simulink model "systemIdentification"  (R2018a)
settings: Solver=FixedStepDiscrete  StartTime=0.0  StopTime=finalTime  FixedStep=sampleTime  RelTol=1e-3
values from neighbouring files (symbols this model uses):
  C1A = 5e-6    (= 5e-06)    [impedance_inductanceAll.m]    (also in impedance_inductancemodel.m)
  C1B = 5e-6    (= 5e-06)    [impedance_inductanceAll.m]    (also in impedance_inductancemodel.m)
  C1C = 5e-6    (= 5e-06)    [impedance_inductanceAll.m]    (also in impedance_inductancemodel.m)
  ESLA = 3e-15    [analytical.m]    (also in impedance_inductanceAll.m = 1.9e-14; impedance_inductancemodel.m = 1.9e-14)
  ESLB = 3e-15    [analytical.m]    (also in impedance_inductanceAll.m = 1.9e-14; impedance_inductancemodel.m = 1.9e-14)
  ESLC = 3e-15    [analytical.m]    (also in impedance_inductanceAll.m = 1.9e-14; impedance_inductancemodel.m = 1.9e-14)
  LA = 0.0150    (= 0.015)    [impedance_inductanceAll.m]
  LABBot = 3e-9    (= 3e-09)    [analytical.m]    (also in impedance_inductanceAll.m = 1.02e-08; impedance_inductancemodel.m = 1.02e-08)
  LABot = 3e-9    (= 3e-09)    [analytical.m]    (also in impedance_inductanceAll.m = 2.025e-08; impedance_inductancemodel.m = 2.025e-08)
  LABTop = 3e-9    (= 3e-09)    [analytical.m]    (also in impedance_inductanceAll.m = 1.83e-08; impedance_inductancemodel.m = 1.83e-08)
  LAMid = 01.30e-9    (= 1.3e-09)    [impedance_inductanceAll.m]    (also in impedance_inductancemodel.m)
  LATop = 3e-9    (= 3e-09)    [analytical.m]    (also in impedance_inductanceAll.m = 3.4e-09; impedance_inductancemodel.m = 3.4e-09)
  LB = 0.0150    (= 0.015)    [impedance_inductanceAll.m]
  LBBot = 3e-9    (= 3e-09)    [analytical.m]    (also in impedance_inductanceAll.m = 2.038e-08; impedance_inductancemodel.m = 2.038e-08)
  LBCBot = 3e-9    (= 3e-09)    [analytical.m]    (also in impedance_inductanceAll.m = 1.114e-08; impedance_inductancemodel.m = 1.114e-08)
  LBCTop = 3e-9    (= 3e-09)    [analytical.m]    (also in impedance_inductanceAll.m = 2.184e-08; impedance_inductancemodel.m = 2.184e-08)
  LBMid = 01.30e-9    (= 1.3e-09)    [impedance_inductanceAll.m]    (also in impedance_inductancemodel.m)
  LBTop = 3e-9    (= 3e-09)    [analytical.m]    (also in impedance_inductanceAll.m = 3.38e-09; impedance_inductancemodel.m = 3.38e-09)
  LC = 0.0150    (= 0.015)    [impedance_inductanceAll.m]
  LCBot = 3e-9    (= 3e-09)    [analytical.m]    (also in impedance_inductanceAll.m = 2.094e-08; impedance_inductancemodel.m = 2.094e-08)
  LCMid = 01.30e-9    (= 1.3e-09)    [impedance_inductanceAll.m]    (also in impedance_inductancemodel.m)
  LCTop = 3e-9    (= 3e-09)    [analytical.m]    (also in impedance_inductanceAll.m = 3.41e-09; impedance_inductancemodel.m = 3.41e-09)
  RA = 10    [impedance_inductanceAll.m]
  RB = 10    [impedance_inductanceAll.m]
  RC = 10    [impedance_inductanceAll.m]
  sampleTime = 1e-7    (= 1e-07)    [impedance_inductanceAll.m]
libraries: powerlib x30, dspsrcs4 x1
settings Model: Creator=enes_  LastModifiedBy=enes_

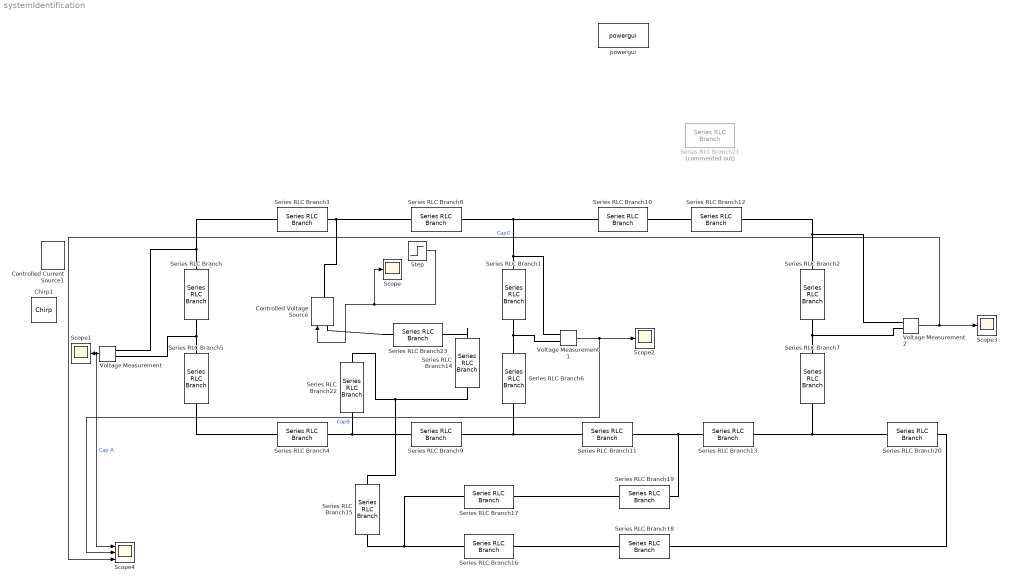
== system systemIdentification ==
  Chirp1 : dspsrcs4/Chirp  sweep=Linear  mode=Unidirectional  f0=0  f1=400000  t1=1  Tsweep=1  phase=0  Ts=sampleTime  spf=1  datatype=Double  OutputFrames=off
      settings: SourceProductName=DSP System Toolbox
  Controlled Current Source1 : powerlib/Electrical Sources/Controlled Current Source  Initialize=on  Source_Type=AC  Amplitude=0  Phase=0  Frequency=0  Measurements=None
  Controlled Voltage Source : powerlib/Electrical Sources/Controlled Voltage Source  Initialize=on  Source_Type=AC  Amplitude=0  Phase=0  Frequency=0  Measurements=None
  Scope{,1..3} (4 alike) : Scope
  Scope4 : Scope  NumInputPorts=3
  Series RLC Branch : powerlib/Elements/Series RLC Branch  LConnTagsString=__new0  RConnTagsString=__new0  BranchType=C  Resistance=1  Inductance=1e-3  SetiL0=off  InitialCurrent=0  Capacitance=C1A  Setx0=off  InitialVoltage=0  Measurements=None
  Series RLC Branch1 : powerlib/Elements/Series RLC Branch  LConnTagsString=__new0  RConnTagsString=__new0  BranchType=C  Resistance=1  Inductance=1e-3  SetiL0=off  InitialCurrent=0  Capacitance=C1B  Setx0=off  InitialVoltage=0  Measurements=None
  Series RLC Branch10 : powerlib/Elements/Series RLC Branch  LConnTagsString=__new0  RConnTagsString=__new0  BranchType=L  Resistance=1  Inductance=LBTop  SetiL0=off  InitialCurrent=0  Capacitance=1e-6  Setx0=off  InitialVoltage=0  Measurements=None
  Series RLC Branch11 : powerlib/Elements/Series RLC Branch  LConnTagsString=__new0  RConnTagsString=__new0  BranchType=L  Resistance=1  Inductance=LBBot  SetiL0=off  InitialCurrent=0  Capacitance=1e-6  Setx0=off  InitialVoltage=0  Measurements=None
  Series RLC Branch12 : powerlib/Elements/Series RLC Branch  LConnTagsString=__new0  RConnTagsString=__new0  BranchType=L  Resistance=1  Inductance=LBCTop  SetiL0=off  InitialCurrent=0  Capacitance=1e-6  Setx0=off  InitialVoltage=0  Measurements=None
  Series RLC Branch13 : powerlib/Elements/Series RLC Branch  LConnTagsString=__new0  RConnTagsString=__new0  BranchType=L  Resistance=1  Inductance=LBCBot  SetiL0=off  InitialCurrent=0  Capacitance=1e-6  Setx0=off  InitialVoltage=0  Measurements=None
  Series RLC Branch14 : powerlib/Elements/Series RLC Branch  LConnTagsString=__new0  RConnTagsString=__new0  BranchType=L  Resistance=1  Inductance=LAMid/2  SetiL0=off  InitialCurrent=0  Capacitance=1e-6  Setx0=off  InitialVoltage=0  Measurements=None
  Series RLC Branch15 : powerlib/Elements/Series RLC Branch  LConnTagsString=__new0  RConnTagsString=__new0  BranchType=RL  Resistance=RA  Inductance=LA  SetiL0=off  InitialCurrent=0  Capacitance=1e-6  Setx0=off  InitialVoltage=0  Measurements=None
  Series RLC Branch16 : powerlib/Elements/Series RLC Branch  LConnTagsString=__new0  RConnTagsString=__new0  BranchType=RL  Resistance=RC  Inductance=LC  SetiL0=off  InitialCurrent=0  Capacitance=1e-6  Setx0=off  InitialVoltage=0  Measurements=None
  Series RLC Branch17 : powerlib/Elements/Series RLC Branch  LConnTagsString=__new0  RConnTagsString=__new0  BranchType=RL  Resistance=RB  Inductance=LB  SetiL0=off  InitialCurrent=0  Capacitance=1e-6  Setx0=off  InitialVoltage=0  Measurements=None
  Series RLC Branch18 : powerlib/Elements/Series RLC Branch  LConnTagsString=__new0  RConnTagsString=__new0  BranchType=L  Resistance=1  Inductance=LCMid/2  SetiL0=off  InitialCurrent=0  Capacitance=1e-6  Setx0=off  InitialVoltage=0  Measurements=None
  Series RLC Branch19 : powerlib/Elements/Series RLC Branch  LConnTagsString=__new0  RConnTagsString=__new0  BranchType=L  Resistance=1  Inductance=LBMid/2  SetiL0=off  InitialCurrent=0  Capacitance=1e-6  Setx0=off  InitialVoltage=0  Measurements=None
  Series RLC Branch2 : powerlib/Elements/Series RLC Branch  LConnTagsString=__new0  RConnTagsString=__new0  BranchType=C  Resistance=1  Inductance=1e-3  SetiL0=off  InitialCurrent=0  Capacitance=C1C  Setx0=off  InitialVoltage=0  Measurements=None
  Series RLC Branch20 : powerlib/Elements/Series RLC Branch  LConnTagsString=__new0  RConnTagsString=__new0  BranchType=L  Resistance=1  Inductance=LCBot  SetiL0=off  InitialCurrent=0  Capacitance=1e-6  Setx0=off  InitialVoltage=0  Measurements=None
  Series RLC Branch21 : powerlib/Elements/Series RLC Branch  Commented=on  LConnTagsString=__new0  RConnTagsString=__new0  BranchType=L  Resistance=1  Inductance=LCTop  SetiL0=off  InitialCurrent=0  Capacitance=1e-6  Setx0=off  InitialVoltage=0  Measurements=None
  Series RLC Branch22 : powerlib/Elements/Series RLC Branch  LConnTagsString=__new0  RConnTagsString=__new0  BranchType=L  Resistance=1  Inductance=LAMid/2  SetiL0=off  InitialCurrent=0  Capacitance=1e-6  Setx0=off  InitialVoltage=0  Measurements=None
  Series RLC Branch23 : powerlib/Elements/Series RLC Branch  LConnTagsString=__new0  RConnTagsString=__new0  BranchType=R  Resistance=0.01  Inductance=LBTop  SetiL0=off  InitialCurrent=0  Capacitance=1e-6  Setx0=off  InitialVoltage=0  Measurements=None
  Series RLC Branch3 : powerlib/Elements/Series RLC Branch  LConnTagsString=__new0  RConnTagsString=__new0  BranchType=L  Resistance=1  Inductance=LATop  SetiL0=off  InitialCurrent=0  Capacitance=1e-6  Setx0=off  InitialVoltage=0  Measurements=None
  Series RLC Branch4 : powerlib/Elements/Series RLC Branch  LConnTagsString=__new0  RConnTagsString=__new0  BranchType=L  Resistance=1  Inductance=LABot  SetiL0=off  InitialCurrent=0  Capacitance=1e-6  Setx0=off  InitialVoltage=0  Measurements=None
  Series RLC Branch5 : powerlib/Elements/Series RLC Branch  LConnTagsString=__new0  RConnTagsString=__new0  BranchType=L  Resistance=1  Inductance=ESLA  SetiL0=off  InitialCurrent=0  Capacitance=1e-6  Setx0=off  InitialVoltage=0  Measurements=None
  Series RLC Branch6 : powerlib/Elements/Series RLC Branch  LConnTagsString=__new0  RConnTagsString=__new0  BranchType=L  Resistance=1  Inductance=ESLB  SetiL0=off  InitialCurrent=0  Capacitance=1e-6  Setx0=off  InitialVoltage=0  Measurements=None
  Series RLC Branch7 : powerlib/Elements/Series RLC Branch  LConnTagsString=__new0  RConnTagsString=__new0  BranchType=L  Resistance=1  Inductance=ESLC  SetiL0=off  InitialCurrent=0  Capacitance=1e-6  Setx0=off  InitialVoltage=0  Measurements=None
  Series RLC Branch8 : powerlib/Elements/Series RLC Branch  LConnTagsString=__new0  RConnTagsString=__new0  BranchType=L  Resistance=1  Inductance=LABTop  SetiL0=off  InitialCurrent=0  Capacitance=1e-6  Setx0=off  InitialVoltage=0  Measurements=None
  Series RLC Branch9 : powerlib/Elements/Series RLC Branch  LConnTagsString=__new0  RConnTagsString=__new0  BranchType=L  Resistance=1  Inductance=LABBot  SetiL0=off  InitialCurrent=0  Capacitance=1e-6  Setx0=off  InitialVoltage=0  Measurements=None
  Step : Step  Time=0.1e-3  SampleTime=0
  Voltage Measurement : powerlib/Measurements/Voltage Measurement  PhasorSimulation=off  OutputType=Complex  PSBequivalent=0
  Voltage Measurement1 : powerlib/Measurements/Voltage Measurement  PhasorSimulation=off  OutputType=Complex  PSBequivalent=0
  Voltage Measurement2 : powerlib/Measurements/Voltage Measurement  PhasorSimulation=off  OutputType=Complex  PSBequivalent=0
  powergui : powerlib/powergui  Priority=1  SimulationMode=Discrete  SampleTime=sampleTime  frequency=60  Iterations=50  frequencyindice=0  Pbase=100e6  ErrMax=1e-4  UnitsV=kV  UnitsW=MW  buscounter=0  FunctionMessages=off  echomessages=off  EnableUseOfTLC=off  CurrentSourceSwitches=off  DisableSnubberDevices=off  DisableRonSwitches=off  DisableVfSwitches=off  DisplayEquations=off  SolverType=Tustin/Backward Euler (TBE)  Interpol=off  ExternalGateDelay=off  methode=off  Ts=100  x0status=blocks  SPID=on  SwTol=0  HookPort=off  RestoreLinks=warning  ResistiveCurrentMeasurement=off  Frange=[0:2:500]  Ylog=off  Xlog=on  ShowGrid=off  save=off  variable=ZData  structure=ScopeData1  ZoomFFT=off  StartTime=0  cycles=1  DisplayStyle=5  fundamental=10000  FreqAxis=off  MaxFrequency=1000000  frequencyindicesteady=1  RmsSteady=1  display=off
  wires:
  Step/1 -> Scope/1, Controlled Voltage Source/1
  Voltage Measurement/1 -> Scope4/1, Scope1/1  "Cap A"
  Voltage Measurement1/1 -> Scope4/2, Scope2/1  "CapB"
  Voltage Measurement2/1 -> Scope4/3, Scope3/1  "CapC"
  connections:
  Series RLC Branch5/LConn1 -- Voltage Measurement/LConn2 -- Series RLC Branch/RConn1
  Series RLC Branch6/LConn1 -- Voltage Measurement1/LConn2 -- Series RLC Branch1/RConn1
  Series RLC Branch7/LConn1 -- Voltage Measurement2/LConn2 -- Series RLC Branch2/RConn1
  Series RLC Branch3/LConn1 -- Voltage Measurement/LConn1 -- Series RLC Branch/LConn1
  Series RLC Branch5/RConn1 -- Series RLC Branch4/LConn1
  Series RLC Branch8/LConn1 -- Controlled Voltage Source/RConn1 -- Series RLC Branch3/RConn1
  Series RLC Branch8/RConn1 -- Series RLC Branch10/LConn1 -- Voltage Measurement1/LConn1 -- Series RLC Branch1/LConn1
  Series RLC Branch4/RConn1 -- Series RLC Branch22/RConn1 -- Series RLC Branch9/LConn1
  Series RLC Branch9/RConn1 -- Series RLC Branch11/LConn1 -- Series RLC Branch6/RConn1
  Series RLC Branch12/LConn1 -- Series RLC Branch10/RConn1
  Series RLC Branch12/RConn1 -- Voltage Measurement2/LConn1 -- Series RLC Branch2/LConn1
  Series RLC Branch11/RConn1 -- Series RLC Branch19/LConn1 -- Series RLC Branch13/LConn1
  Series RLC Branch13/RConn1 -- Series RLC Branch20/LConn1 -- Series RLC Branch7/RConn1
  Series RLC Branch23/LConn1 -- Controlled Voltage Source/LConn1
  Series RLC Branch14/RConn1 -- Series RLC Branch22/LConn1 -- Series RLC Branch15/LConn1
  Series RLC Branch16/LConn1 -- Series RLC Branch17/LConn1 -- Series RLC Branch15/RConn1
  Series RLC Branch16/RConn1 -- Series RLC Branch18/RConn1
  Series RLC Branch19/RConn1 -- Series RLC Branch17/RConn1
  Series RLC Branch18/LConn1 -- Series RLC Branch20/RConn1
  Series RLC Branch14/LConn1 -- Series RLC Branch23/RConn1
